simulink model "project_model"  (R2021b)
settings: Solver=VariableStepAuto  StartTime=0.0  StopTime=10.0  RelTol=1e-3
undefined symbols (not defined in the file): K
settings Model: Creator=Reyhaneh  LastModifiedBy=Reyhaneh

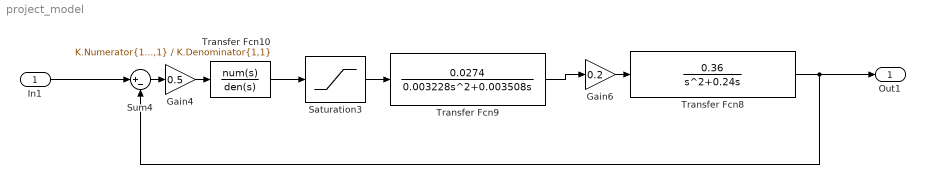
== system project_model ==
  In1 : Inport
  Gain4 : Gain  Gain=0.5
  Gain6 : Gain  Gain=0.2
  Saturation3 : Saturate  UpperLimit=20  LowerLimit=-20
  Sum4 : Sum  Inputs=|+-
  Transfer Fcn10 : TransferFcn  Numerator=K.Numerator{1,1}  Denominator=K.Denominator{1,1}
  Transfer Fcn8 : TransferFcn  Numerator=[0.36]  Denominator=[1 0.24 0]
  Transfer Fcn9 : TransferFcn  Numerator=[0.0274]  Denominator=[0.003228 0.003508 0]
  Out1 : Outport
  wires:
  Transfer Fcn8/1 -> Out1/1, Sum4/2
  Transfer Fcn9/1 -> Gain6/1
  Transfer Fcn10/1 -> Saturation3/1
  Gain4/1 -> Transfer Fcn10/1
  Saturation3/1 -> Transfer Fcn9/1
  In1/1 -> Sum4/1
  Gain6/1 -> Transfer Fcn8/1
  Sum4/1 -> Gain4/1
